simulink model "ModeStatAndRsp_2"  (R2018b)
settings: Solver=FixedStepDiscrete  StartTime=0.0  StopTime=10.0  FixedStep=0.01  RelTol=1e-3
settings Model: Creator=sn2xws  LastModifiedBy=sn2xws
settings ModelReferenceCC: ModelReferenceNumInstancesAllowed=Single

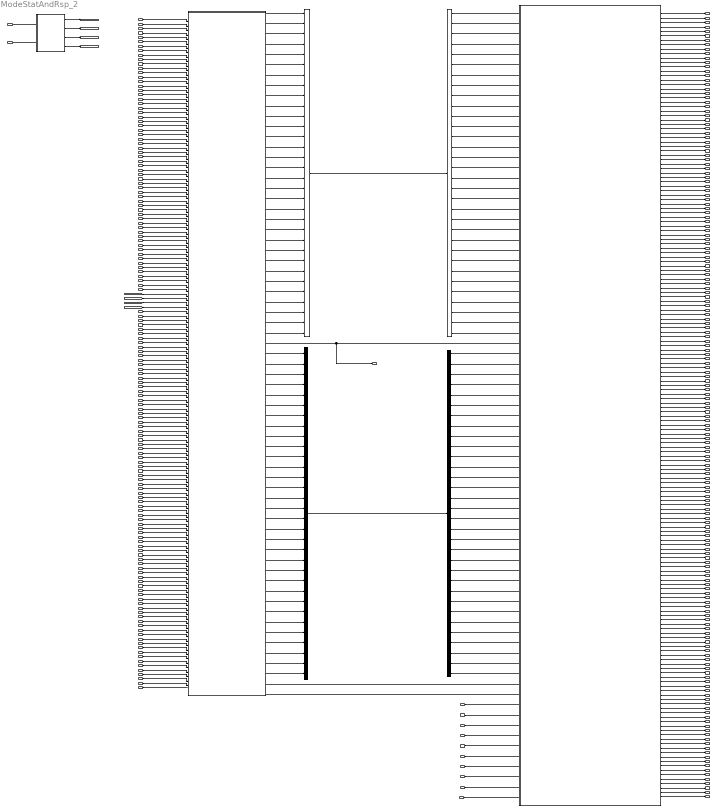
== system ModeStatAndRsp_2 ==
  MdXX_isTrgtPosRunnable : Inport  SampleTime=0.01  OutputFunctionCall=on
  isAcsMdEntryArrivedAtTargetPos_Val : Inport  Port=2  OutDataTypeStr=boolean  PortDimensions=1
  isAcsMdExtArrivedAtTargetPos_Val : Inport  Port=3  OutDataTypeStr=boolean  PortDimensions=1
  isINTMArrivedAtTargetPos_Val : Inport  Port=4  OutDataTypeStr=boolean  PortDimensions=1
  isINTMRArrivedAtTargetPos_Val : Inport  Port=5  OutDataTypeStr=boolean  PortDimensions=1
  isLfFamlyArrivedAtTargetPos_Val : Inport  Port=6  OutDataTypeStr=boolean  PortDimensions=1
  isLfLugArrivedAtTargetPos_Val : Inport  Port=7  OutDataTypeStr=boolean  PortDimensions=1
  isLfLyArrivedAtTargetPos_Val : Inport  Port=8  OutDataTypeStr=boolean  PortDimensions=1
  isLfRecoveryArrivedAtTargetPos_Val : Inport  Port=9  OutDataTypeStr=boolean  PortDimensions=1
  isLfVipArrivedAtTargetPos_Val : Inport  Port=10  OutDataTypeStr=boolean  PortDimensions=1
  isLgrstCloseLArrivedAtTargetPos_Val : Inport  Port=11  OutDataTypeStr=boolean  PortDimensions=1
  isLgrstCloseRArrivedAtTargetPos_Val : Inport  Port=12  OutDataTypeStr=boolean  PortDimensions=1
  isLgrstOpenLArrivedAtTargetPos_Val : Inport  Port=13  OutDataTypeStr=boolean  PortDimensions=1
  isLgrstOpenRArrivedAtTargetPos_Val : Inport  Port=14  OutDataTypeStr=boolean  PortDimensions=1
  isRtFamlyArrivedAtTargetPos_Val : Inport  Port=15  OutDataTypeStr=boolean  PortDimensions=1
  isRtLugArrivedAtTargetPos_Val : Inport  Port=16  OutDataTypeStr=boolean  PortDimensions=1
  isRtLyArrivedAtTargetPos_Val : Inport  Port=17  OutDataTypeStr=boolean  PortDimensions=1
  isRtRecoveryArrivedAtTargetPos_Val : Inport  Port=18  OutDataTypeStr=boolean  PortDimensions=1
  isRtVipArrivedAtTargetPos_Val : Inport  Port=19  OutDataTypeStr=boolean  PortDimensions=1
  MdXX_RspOutCommRunnable : Inport  Port=20  SampleTime=0.01  OutputFunctionCall=on
  MdXX_StatusRunnable : Inport  Port=21  SampleTime=0.01  OutputFunctionCall=on
  StPassCmprtMdHMIDisCmdRunnable : Inport  Port=22  SampleTime=0.01  OutputFunctionCall=on
  PwrMdChked_Val : Inport  Port=23  OutDataTypeStr=Enum: PowerMode1  PortDimensions=1
  CHM2CtrlRunnable : Inport  Port=24  SampleTime=0.01  OutputFunctionCall=on
  IfVeSMSuChmMgrStat_Val : Inport  Port=25  OutDataTypeStr=uint16  PortDimensions=1
  MdXX_StatusToNetWorkRunnable : Inport  Port=26  SampleTime=0.01  OutputFunctionCall=on
  MdXX_RspSelcRunnable : Inport  Port=27  SampleTime=0.01  OutputFunctionCall=on
  SRSModeStateRunnable : Inport  Port=28  SampleTime=0.01  OutputFunctionCall=on
  StNumChkRunnable : Inport  Port=29  SampleTime=0.01  OutputFunctionCall=on
  IfVeSMSeStNumConfig_Val : Inport  Port=30  OutDataTypeStr=Enum: IfVeSMSeStNumConfig  PortDimensions=1
  StateOnOffChkRunnable : Inport  Port=31  SampleTime=0.01  OutputFunctionCall=on
  CommCond_Val : Inport  Port=32  OutDataTypeStr=boolean  PortDimensions=1
  CommExitCond_Val : Inport  Port=33  OutDataTypeStr=boolean  PortDimensions=1
  CommExitCondwithSpeed_Val : Inport  Port=34  OutDataTypeStr=boolean  PortDimensions=1
  isAcsMdEntryDoneFailed_Val : Inport  Port=35  OutDataTypeStr=boolean  PortDimensions=1
  isAcsMdEntryDoneOK_Val : Inport  Port=36  OutDataTypeStr=boolean  PortDimensions=1
  isAcsMdExtDoneFailed_Val : Inport  Port=37  OutDataTypeStr=boolean  PortDimensions=1
  isAcsMdExtDoneOK_Val : Inport  Port=38  OutDataTypeStr=boolean  PortDimensions=1
  isINTMDoneFailed_Val : Inport  Port=39  OutDataTypeStr=boolean  PortDimensions=1
  isINTMDoneOK_Val : Inport  Port=40  OutDataTypeStr=boolean  PortDimensions=1
  isINTMRDoneFailed_Val : Inport  Port=41  OutDataTypeStr=boolean  PortDimensions=1
  isINTMRDoneOK_Val : Inport  Port=42  OutDataTypeStr=boolean  PortDimensions=1
  isLfFamlyDoneFailed_Val : Inport  Port=43  OutDataTypeStr=boolean  PortDimensions=1
  isLfFamlyDoneOK_Val : Inport  Port=44  OutDataTypeStr=boolean  PortDimensions=1
  isLfLugDoneFailed_Val : Inport  Port=45  OutDataTypeStr=boolean  PortDimensions=1
  isLfLugDoneOK_Val : Inport  Port=46  OutDataTypeStr=boolean  PortDimensions=1
  isLfLyDoneFailed_Val : Inport  Port=47  OutDataTypeStr=boolean  PortDimensions=1
  isLfLyDoneOK_Val : Inport  Port=48  OutDataTypeStr=boolean  PortDimensions=1
  isLfRecoveryDoneFailed_Val : Inport  Port=49  OutDataTypeStr=boolean  PortDimensions=1
  isLfRecoveryDoneOK_Val : Inport  Port=50  OutDataTypeStr=boolean  PortDimensions=1
  isLfVipDoneFailed_Val : Inport  Port=51  OutDataTypeStr=boolean  PortDimensions=1
  isLfVipDoneOK_Val : Inport  Port=52  OutDataTypeStr=boolean  PortDimensions=1
  isLgrstCloseLDoneFailed_Val : Inport  Port=53  OutDataTypeStr=boolean  PortDimensions=1
  isLgrstCloseLDoneOK_Val : Inport  Port=54  OutDataTypeStr=boolean  PortDimensions=1
  isLgrstCloseRDoneFailed_Val : Inport  Port=55  OutDataTypeStr=boolean  PortDimensions=1
  isLgrstCloseRDoneOK_Val : Inport  Port=56  OutDataTypeStr=boolean  PortDimensions=1
  isLgrstOpenLDoneFailed_Val : Inport  Port=57  OutDataTypeStr=boolean  PortDimensions=1
  isLgrstOpenLDoneOK_Val : Inport  Port=58  OutDataTypeStr=boolean  PortDimensions=1
  isLgrstOpenRDoneFailed_Val : Inport  Port=59  OutDataTypeStr=boolean  PortDimensions=1
  isLgrstOpenRDoneOK_Val : Inport  Port=60  OutDataTypeStr=boolean  PortDimensions=1
  isRfFamlyDoneFailed_Val : Inport  Port=61  OutDataTypeStr=boolean  PortDimensions=1
  isRfFamlyDoneOK_Val : Inport  Port=62  OutDataTypeStr=boolean  PortDimensions=1
  isRtLugDoneFailed_Val : Inport  Port=63  OutDataTypeStr=boolean  PortDimensions=1
  isRtLugDoneOK_Val : Inport  Port=64  OutDataTypeStr=boolean  PortDimensions=1
  isRtLyDoneFailed_Val : Inport  Port=65  OutDataTypeStr=boolean  PortDimensions=1
  isRtLyDoneOK_Val : Inport  Port=66  OutDataTypeStr=boolean  PortDimensions=1
  isRtRecoveryDoneFailed_Val : Inport  Port=67  OutDataTypeStr=boolean  PortDimensions=1
  isRtRecoveryDoneOK_Val : Inport  Port=68  OutDataTypeStr=boolean  PortDimensions=1
  isRtVipDoneFailed_Val : Inport  Port=69  OutDataTypeStr=boolean  PortDimensions=1
  isRtVipDoneOK_Val : Inport  Port=70  OutDataTypeStr=boolean  PortDimensions=1
  R3LMdSeatOccupied_Val : Inport  Port=71  OutDataTypeStr=boolean  PortDimensions=1
  R3RMdSeatOccupied_Val : Inport  Port=72  OutDataTypeStr=boolean  PortDimensions=1
  SoftIntAcsEnty_Val : Inport  Port=73  OutDataTypeStr=IntEnable  PortDimensions=1
  SoftIntAcsExt_Val : Inport  Port=74  OutDataTypeStr=IntEnable  PortDimensions=1
  SoftIntAllLug_Val : Inport  Port=75  OutDataTypeStr=IntEnable  PortDimensions=1
  SoftIntAllVip_Val : Inport  Port=76  OutDataTypeStr=IntEnable  PortDimensions=1
  SoftIntIntimacyRt_Val : Inport  Port=77  OutDataTypeStr=IntEnable  PortDimensions=1
  SoftIntINTM_Val : Inport  Port=78  OutDataTypeStr=IntEnable  PortDimensions=1
  SoftIntLfFamly_Val : Inport  Port=79  OutDataTypeStr=IntEnable  PortDimensions=1
  SoftIntLfLug_Val : Inport  Port=80  OutDataTypeStr=IntEnable  PortDimensions=1
  SoftIntLfLy_Val : Inport  Port=81  OutDataTypeStr=IntEnable  PortDimensions=1
  SoftIntLfRcvy_Val : Inport  Port=82  OutDataTypeStr=IntEnable  PortDimensions=1
  SoftIntLfVip_Val : Inport  Port=83  OutDataTypeStr=IntEnable  PortDimensions=1
  SoftIntLgrstCloseLt_Val : Inport  Port=84  OutDataTypeStr=IntEnable  PortDimensions=1
  SoftIntLgrstCloseRt_Val : Inport  Port=85  OutDataTypeStr=IntEnable  PortDimensions=1
  SoftIntLgrstOpenLt_Val : Inport  Port=86  OutDataTypeStr=IntEnable  PortDimensions=1
  SoftIntLgrstOpenRt_Val : Inport  Port=87  OutDataTypeStr=IntEnable  PortDimensions=1
  SoftIntRtFamly_Val : Inport  Port=88  OutDataTypeStr=IntEnable  PortDimensions=1
  SoftIntRtLug_Val : Inport  Port=89  OutDataTypeStr=IntEnable  PortDimensions=1
  SoftIntRtLy_Val : Inport  Port=90  OutDataTypeStr=IntEnable  PortDimensions=1
  SoftIntRtRcvy_Val : Inport  Port=91  OutDataTypeStr=IntEnable  PortDimensions=1
  SoftIntRtVip_Val : Inport  Port=92  OutDataTypeStr=IntEnable  PortDimensions=1
  SwIntAcsEnty_Val : Inport  Port=93  OutDataTypeStr=IntEnable  PortDimensions=1
  SwIntAcsExt_Val : Inport  Port=94  OutDataTypeStr=IntEnable  PortDimensions=1
  SwIntAllLug_Val : Inport  Port=95  OutDataTypeStr=IntEnable  PortDimensions=1
  SwIntAllVip_Val : Inport  Port=96  OutDataTypeStr=IntEnable  PortDimensions=1
  SwIntIntimacyRt_Val : Inport  Port=97  OutDataTypeStr=IntEnable  PortDimensions=1
  SwIntINTM_Val : Inport  Port=98  OutDataTypeStr=IntEnable  PortDimensions=1
  SwIntLfFamly_Val : Inport  Port=99  OutDataTypeStr=IntEnable  PortDimensions=1
  SwIntLfLug_Val : Inport  Port=100  OutDataTypeStr=IntEnable  PortDimensions=1
  SwIntLfLy_Val : Inport  Port=101  OutDataTypeStr=IntEnable  PortDimensions=1
  SwIntLfRcvy_Val : Inport  Port=102  OutDataTypeStr=IntEnable  PortDimensions=1
  SwIntLfVip_Val : Inport  Port=103  OutDataTypeStr=IntEnable  PortDimensions=1
  SwIntLgrstCloseLt_Val : Inport  Port=104  OutDataTypeStr=IntEnable  PortDimensions=1
  SwIntLgrstCloseRt_Val : Inport  Port=105  OutDataTypeStr=IntEnable  PortDimensions=1
  SwIntLgrstOpenLt_Val : Inport  Port=106  OutDataTypeStr=IntEnable  PortDimensions=1
  SwIntLgrstOpenRt_Val : Inport  Port=107  OutDataTypeStr=IntEnable  PortDimensions=1
  SwIntRtFamly_Val : Inport  Port=108  OutDataTypeStr=IntEnable  PortDimensions=1
  SwIntRtLug_Val : Inport  Port=109  OutDataTypeStr=IntEnable  PortDimensions=1
  SwIntRtLy_Val : Inport  Port=110  OutDataTypeStr=IntEnable  PortDimensions=1
  SwIntRtRcvy_Val : Inport  Port=111  OutDataTypeStr=IntEnable  PortDimensions=1
  SwIntRtVip_Val : Inport  Port=112  OutDataTypeStr=IntEnable  PortDimensions=1
  MdXX_RspChkRunnable : Inport  Port=113  SampleTime=0.01  OutputFunctionCall=on
  acsEntyMdReq_Val : Inport  Port=114  OutDataTypeStr=boolean  PortDimensions=1
  acsExtMdReq_Val : Inport  Port=115  OutDataTypeStr=boolean  PortDimensions=1
  AllLugMdReq_Val : Inport  Port=116  OutDataTypeStr=boolean  PortDimensions=1
  AllVipMdReq_Val : Inport  Port=117  OutDataTypeStr=boolean  PortDimensions=1
  IntimacyRtMdReq_Val : Inport  Port=118  OutDataTypeStr=boolean  PortDimensions=1
  INTMMdReq_Val : Inport  Port=119  OutDataTypeStr=boolean  PortDimensions=1
  LfFamlyReq_Val : Inport  Port=120  OutDataTypeStr=boolean  PortDimensions=1
  LfLyMdReq_Val : Inport  Port=121  OutDataTypeStr=boolean  PortDimensions=1
  LgrstCloseLtMdReq_Val : Inport  Port=122  OutDataTypeStr=boolean  PortDimensions=1
  LgrstCloseRtMdReq_Val : Inport  Port=123  OutDataTypeStr=boolean  PortDimensions=1
  LgrstOpenLtMdReq_Val : Inport  Port=124  OutDataTypeStr=boolean  PortDimensions=1
  LgrstOpenRtMdReq_Val : Inport  Port=125  OutDataTypeStr=boolean  PortDimensions=1
  LtLugMdReq_Val : Inport  Port=126  OutDataTypeStr=boolean  PortDimensions=1
  LtRcvyMdReq_Val : Inport  Port=127  OutDataTypeStr=boolean  PortDimensions=1
  LtVipMdReq_Val : Inport  Port=128  OutDataTypeStr=boolean  PortDimensions=1
  RtFamlyMdReq_Val : Inport  Port=129  OutDataTypeStr=boolean  PortDimensions=1
  RtLugMdReq_Val : Inport  Port=130  OutDataTypeStr=boolean  PortDimensions=1
  RtLyMdReq_Val : Inport  Port=131  OutDataTypeStr=boolean  PortDimensions=1
  RtRcvyMdReq_Val : Inport  Port=132  OutDataTypeStr=boolean  PortDimensions=1
  RtVipMdReq_Val : Inport  Port=133  OutDataTypeStr=boolean  PortDimensions=1
  LugMdLtAvl_Val : Inport  Port=134  OutDataTypeStr=boolean  PortDimensions=1
  LugMdRtAvl_Val : Inport  Port=135  OutDataTypeStr=boolean  PortDimensions=1
  VipMdLtAvl_Val : Inport  Port=136  OutDataTypeStr=boolean  PortDimensions=1
  VipMdRtAvl_Val : Inport  Port=137  OutDataTypeStr=boolean  PortDimensions=1
  MdEnCtrlAndBsyChkRunnable : Inport  Port=138  SampleTime=0.01  OutputFunctionCall=on
  MdXX_SrcTpRunnable : Inport  Port=139  SampleTime=0.01  OutputFunctionCall=on
  acsEntyMdSrcTp_Val : Inport  Port=140  OutDataTypeStr=Enum: SrcReqTp1  PortDimensions=1
  acsExtMdSrcTp_Val : Inport  Port=141  OutDataTypeStr=Enum: SrcReqTp1  PortDimensions=1
  AllLugSrcReqTp_Val : Inport  Port=142  OutDataTypeStr=Enum: SrcReqTp1  PortDimensions=1
  AllVipSrcReqTp_Val : Inport  Port=143  OutDataTypeStr=Enum: SrcReqTp1  PortDimensions=1
  IntimacyRtMdSrcTp_Val : Inport  Port=144  OutDataTypeStr=Enum: SrcReqTp1  PortDimensions=1
  INTMSrcReqTp_Val : Inport  Port=145  OutDataTypeStr=Enum: SrcReqTp1  PortDimensions=1
  LfFamlySrcReqTp_Val : Inport  Port=146  OutDataTypeStr=Enum: SrcReqTp1  PortDimensions=1
  LfLySrcReqTp_Val : Inport  Port=147  OutDataTypeStr=Enum: SrcReqTp1  PortDimensions=1
  LgrstCloseLtSrcReqTp_Val : Inport  Port=148  OutDataTypeStr=Enum: SrcReqTp1  PortDimensions=1
  LgrstCloseRtSrcReqTp_Val : Inport  Port=149  OutDataTypeStr=Enum: SrcReqTp1  PortDimensions=1
  LgrstOpenLtSrcReqTp_Val : Inport  Port=150  OutDataTypeStr=Enum: SrcReqTp1  PortDimensions=1
  LgrstOpenRtSrcReqTp_Val : Inport  Port=151  OutDataTypeStr=Enum: SrcReqTp1  PortDimensions=1
  LtLugSrcReqTp_Val : Inport  Port=152  OutDataTypeStr=Enum: SrcReqTp1  PortDimensions=1
  LtRcvySrcReqTp_Val : Inport  Port=153  OutDataTypeStr=Enum: SrcReqTp1  PortDimensions=1
  LtVipSrcReqTp_Val : Inport  Port=154  OutDataTypeStr=Enum: SrcReqTp1  PortDimensions=1
  RtFamlySrcReqTp_Val : Inport  Port=155  OutDataTypeStr=Enum: SrcReqTp1  PortDimensions=1
  RtLugSrcReqTp_Val : Inport  Port=156  OutDataTypeStr=Enum: SrcReqTp1  PortDimensions=1
  RtLySrcReqTp_Val : Inport  Port=157  OutDataTypeStr=Enum: SrcReqTp1  PortDimensions=1
  RtRcvySrcReqTp_Val : Inport  Port=158  OutDataTypeStr=Enum: SrcReqTp1  PortDimensions=1
  RtVipSrcReqTp_Val : Inport  Port=159  OutDataTypeStr=Enum: SrcReqTp1  PortDimensions=1
  PosArray_Val : Inport  Port=160  OutDataTypeStr=uint8  PortDimensions=11
  Demux : Demux  Outputs=32
  Demux1 : Demux  Outputs=32
  Model : ModelReference  ModelNameDialog=StNumChk.slx  SimulationMode=Normal  ModelReferenceVersion=V2.0.0
  Model1 : ModelReference  ModelNameDialog=ModeStatCtrl.slx  SimulationMode=Normal  ModelReferenceVersion=1.27
  Model3 : ModelReference  ModelNameDialog=ModeRsp.slx  SimulationMode=Normal  ModelReferenceVersion=1.35
  Mux : Mux  Inputs=32
  Mux1 : Mux  Inputs=32
  IfVeSMSuStPassCmprtMdHMIDisCmd_Val : Outport  OutDataTypeStr=uint8  PortDimensions=1
  IfVeSMSeStPassCmprtMdNoti2ChmEvntStat_Val : Outport  Port=2  OutDataTypeStr=Enum: EventSts1  PortDimensions=1
  IfVeSMSeStPassCmprtMdCrtMdStat_Val : Outport  Port=3  OutDataTypeStr=uint8  PortDimensions=1
  IfVeSMSuStPassCmprtMd_Md1_CrtStat_Val : Outport  Port=4  OutDataTypeStr=uint8  PortDimensions=1
  IfVeSMSuStPassCmprtMd_Md10_CrtStat_Val : Outport  Port=5  OutDataTypeStr=uint8  PortDimensions=1
  IfVeSMSuStPassCmprtMd_Md11_CrtStat_Val : Outport  Port=6  OutDataTypeStr=uint8  PortDimensions=1
  IfVeSMSuStPassCmprtMd_Md12_CrtStat_Val : Outport  Port=7  OutDataTypeStr=uint8  PortDimensions=1
  IfVeSMSuStPassCmprtMd_Md13_CrtStat_Val : Outport  Port=8  OutDataTypeStr=uint8  PortDimensions=1
  IfVeSMSuStPassCmprtMd_Md14_CrtStat_Val : Outport  Port=9  OutDataTypeStr=uint8  PortDimensions=1
  IfVeSMSuStPassCmprtMd_Md15_CrtStat_Val : Outport  Port=10  OutDataTypeStr=uint8  PortDimensions=1
  IfVeSMSuStPassCmprtMd_Md16_CrtStat_Val : Outport  Port=11  OutDataTypeStr=uint8  PortDimensions=1
  IfVeSMSuStPassCmprtMd_Md17_CrtStat_Val : Outport  Port=12  OutDataTypeStr=uint8  PortDimensions=1
  IfVeSMSuStPassCmprtMd_Md18_CrtStat_Val : Outport  Port=13  OutDataTypeStr=uint8  PortDimensions=1
  IfVeSMSuStPassCmprtMd_Md19_CrtStat_Val : Outport  Port=14  OutDataTypeStr=uint8  PortDimensions=1
  IfVeSMSuStPassCmprtMd_Md2_CrtStat_Val : Outport  Port=15  OutDataTypeStr=uint8  PortDimensions=1
  IfVeSMSuStPassCmprtMd_Md20_CrtStat_Val : Outport  Port=16  OutDataTypeStr=uint8  PortDimensions=1
  IfVeSMSuStPassCmprtMd_Md21_CrtStat_Val : Outport  Port=17  OutDataTypeStr=uint8  PortDimensions=1
  IfVeSMSuStPassCmprtMd_Md22_CrtStat_Val : Outport  Port=18  OutDataTypeStr=uint8  PortDimensions=1
  IfVeSMSuStPassCmprtMd_Md23_CrtStat_Val : Outport  Port=19  OutDataTypeStr=uint8  PortDimensions=1
  IfVeSMSuStPassCmprtMd_Md24_CrtStat_Val : Outport  Port=20  OutDataTypeStr=uint8  PortDimensions=1
  IfVeSMSuStPassCmprtMd_Md25_CrtStat_Val : Outport  Port=21  OutDataTypeStr=uint8  PortDimensions=1
  IfVeSMSuStPassCmprtMd_Md26_CrtStat_Val : Outport  Port=22  OutDataTypeStr=uint8  PortDimensions=1
  IfVeSMSuStPassCmprtMd_Md27_CrtStat_Val : Outport  Port=23  OutDataTypeStr=uint8  PortDimensions=1
  IfVeSMSuStPassCmprtMd_Md28_CrtStat_Val : Outport  Port=24  OutDataTypeStr=uint8  PortDimensions=1
  IfVeSMSuStPassCmprtMd_Md29_CrtStat_Val : Outport  Port=25  OutDataTypeStr=uint8  PortDimensions=1
  IfVeSMSuStPassCmprtMd_Md3_CrtStat_Val : Outport  Port=26  OutDataTypeStr=uint8  PortDimensions=1
  IfVeSMSuStPassCmprtMd_Md30_CrtStat_Val : Outport  Port=27  OutDataTypeStr=uint8  PortDimensions=1
  IfVeSMSuStPassCmprtMd_Md31_CrtStat_Val : Outport  Port=28  OutDataTypeStr=uint8  PortDimensions=1
  IfVeSMSuStPassCmprtMd_Md32_CrtStat_Val : Outport  Port=29  OutDataTypeStr=uint8  PortDimensions=1
  IfVeSMSuStPassCmprtMd_Md4_CrtStat_Val : Outport  Port=30  OutDataTypeStr=uint8  PortDimensions=1
  IfVeSMSuStPassCmprtMd_Md5_CrtStat_Val : Outport  Port=31  OutDataTypeStr=uint8  PortDimensions=1
  IfVeSMSuStPassCmprtMd_Md6_CrtStat_Val : Outport  Port=32  OutDataTypeStr=uint8  PortDimensions=1
  IfVeSMSuStPassCmprtMd_Md7_CrtStat_Val : Outport  Port=33  OutDataTypeStr=uint8  PortDimensions=1
  IfVeSMSuStPassCmprtMd_Md8_CrtStat_Val : Outport  Port=34  OutDataTypeStr=uint8  PortDimensions=1
  IfVeSMSuStPassCmprtMd_Md9_CrtStat_Val : Outport  Port=35  OutDataTypeStr=uint8  PortDimensions=1
  IfVeSMSuSRSCrt_MdSw1_Stat_Val : Outport  Port=36  OutDataTypeStr=uint8  PortDimensions=1
  IfVeSMSuSRSCrt_MdSw10_Stat_Val : Outport  Port=37  OutDataTypeStr=uint8  PortDimensions=1
  IfVeSMSuSRSCrt_MdSw2_Stat_Val : Outport  Port=38  OutDataTypeStr=uint8  PortDimensions=1
  IfVeSMSuSRSCrt_MdSw3_Stat_Val : Outport  Port=39  OutDataTypeStr=uint8  PortDimensions=1
  IfVeSMSuSRSCrt_MdSw4_Stat_Val : Outport  Port=40  OutDataTypeStr=uint8  PortDimensions=1
  IfVeSMSuSRSCrt_MdSw5_Stat_Val : Outport  Port=41  OutDataTypeStr=uint8  PortDimensions=1
  IfVeSMSuSRSCrt_MdSw6_Stat_Val : Outport  Port=42  OutDataTypeStr=uint8  PortDimensions=1
  IfVeSMSuSRSCrt_MdSw7_Stat_Val : Outport  Port=43  OutDataTypeStr=uint8  PortDimensions=1
  IfVeSMSuSRSCrt_MdSw8_Stat_Val : Outport  Port=44  OutDataTypeStr=uint8  PortDimensions=1
  IfVeSMSuSRSCrt_MdSw9_Stat_Val : Outport  Port=45  OutDataTypeStr=uint8  PortDimensions=1
  IfVeSMSuSRSCrtMdIndTyp_67_2_Val : Outport  Port=46  OutDataTypeStr=uint8  PortDimensions=1
  IfVeSMStPassCmprtMd_RfCtrl_Sw_RclRspStat_Val : Outport  Port=47  OutDataTypeStr=uint8  PortDimensions=1
  IfVeSMSuHMI2L_StMd1_Rsp_Val : Outport  Port=48  OutDataTypeStr=uint8  PortDimensions=1
  IfVeSMSuHMI2L_StMd10_Rsp_Val : Outport  Port=49  OutDataTypeStr=uint8  PortDimensions=1
  IfVeSMSuHMI2L_StMd11_Rsp_Val : Outport  Port=50  OutDataTypeStr=uint8  PortDimensions=1
  IfVeSMSuHMI2L_StMd12_Rsp_Val : Outport  Port=51  OutDataTypeStr=uint8  PortDimensions=1
  IfVeSMSuHMI2L_StMd13_Rsp_Val : Outport  Port=52  OutDataTypeStr=uint8  PortDimensions=1
  IfVeSMSuHMI2L_StMd14_Rsp_Val : Outport  Port=53  OutDataTypeStr=uint8  PortDimensions=1
  IfVeSMSuHMI2L_StMd15_Rsp_Val : Outport  Port=54  OutDataTypeStr=uint8  PortDimensions=1
  IfVeSMSuHMI2L_StMd16_Rsp_Val : Outport  Port=55  OutDataTypeStr=uint8  PortDimensions=1
  IfVeSMSuHMI2L_StMd17_Rsp_Val : Outport  Port=56  OutDataTypeStr=uint8  PortDimensions=1
  IfVeSMSuHMI2L_StMd18_Rsp_Val : Outport  Port=57  OutDataTypeStr=uint8  PortDimensions=1
  IfVeSMSuHMI2L_StMd19_Rsp_Val : Outport  Port=58  OutDataTypeStr=uint8  PortDimensions=1
  IfVeSMSuHMI2L_StMd2_Rsp_Val : Outport  Port=59  OutDataTypeStr=uint8  PortDimensions=1
  IfVeSMSuHMI2L_StMd20_Rsp_Val : Outport  Port=60  OutDataTypeStr=uint8  PortDimensions=1
  IfVeSMSuHMI2L_StMd21_Rsp_Val : Outport  Port=61  OutDataTypeStr=uint8  PortDimensions=1
  IfVeSMSuHMI2L_StMd22_Rsp_Val : Outport  Port=62  OutDataTypeStr=uint8  PortDimensions=1
  IfVeSMSuHMI2L_StMd23_Rsp_Val : Outport  Port=63  OutDataTypeStr=uint8  PortDimensions=1
  IfVeSMSuHMI2L_StMd24_Rsp_Val : Outport  Port=64  OutDataTypeStr=uint8  PortDimensions=1
  IfVeSMSuHMI2L_StMd25_Rsp_Val : Outport  Port=65  OutDataTypeStr=uint8  PortDimensions=1
  IfVeSMSuHMI2L_StMd26_Rsp_Val : Outport  Port=66  OutDataTypeStr=uint8  PortDimensions=1
  IfVeSMSuHMI2L_StMd27_Rsp_Val : Outport  Port=67  OutDataTypeStr=uint8  PortDimensions=1
  IfVeSMSuHMI2L_StMd28_Rsp_Val : Outport  Port=68  OutDataTypeStr=uint8  PortDimensions=1
  IfVeSMSuHMI2L_StMd29_Rsp_Val : Outport  Port=69  OutDataTypeStr=uint8  PortDimensions=1
  IfVeSMSuHMI2L_StMd3_Rsp_Val : Outport  Port=70  OutDataTypeStr=uint8  PortDimensions=1
  IfVeSMSuHMI2L_StMd30_Rsp_Val : Outport  Port=71  OutDataTypeStr=uint8  PortDimensions=1
  IfVeSMSuHMI2L_StMd31_Rsp_Val : Outport  Port=72  OutDataTypeStr=uint8  PortDimensions=1
  IfVeSMSuHMI2L_StMd32_Rsp_Val : Outport  Port=73  OutDataTypeStr=uint8  PortDimensions=1
  IfVeSMSuHMI2L_StMd4_Rsp_Val : Outport  Port=74  OutDataTypeStr=uint8  PortDimensions=1
  IfVeSMSuHMI2L_StMd5_Rsp_Val : Outport  Port=75  OutDataTypeStr=uint8  PortDimensions=1
  IfVeSMSuHMI2L_StMd6_Rsp_Val : Outport  Port=76  OutDataTypeStr=uint8  PortDimensions=1
  IfVeSMSuHMI2L_StMd7_Rsp_Val : Outport  Port=77  OutDataTypeStr=uint8  PortDimensions=1
  IfVeSMSuHMI2L_StMd8_Rsp_Val : Outport  Port=78  OutDataTypeStr=uint8  PortDimensions=1
  IfVeSMSuHMI2L_StMd9_Rsp_Val : Outport  Port=79  OutDataTypeStr=uint8  PortDimensions=1
  IfVeSMSuHMI2R_StMd1_Rsp_Val : Outport  Port=80  OutDataTypeStr=uint8  PortDimensions=1
  IfVeSMSuHMI2R_StMd10_Rsp_Val : Outport  Port=81  OutDataTypeStr=uint8  PortDimensions=1
  IfVeSMSuHMI2R_StMd11_Rsp_Val : Outport  Port=82  OutDataTypeStr=uint8  PortDimensions=1
  IfVeSMSuHMI2R_StMd12_Rsp_Val : Outport  Port=83  OutDataTypeStr=uint8  PortDimensions=1
  IfVeSMSuHMI2R_StMd13_Rsp_Val : Outport  Port=84  OutDataTypeStr=uint8  PortDimensions=1
  IfVeSMSuHMI2R_StMd14_Rsp_Val : Outport  Port=85  OutDataTypeStr=uint8  PortDimensions=1
  IfVeSMSuHMI2R_StMd15_Rsp_Val : Outport  Port=86  OutDataTypeStr=uint8  PortDimensions=1
  IfVeSMSuHMI2R_StMd16_Rsp_Val : Outport  Port=87  OutDataTypeStr=uint8  PortDimensions=1
  IfVeSMSuHMI2R_StMd17_Rsp_Val : Outport  Port=88  OutDataTypeStr=uint8  PortDimensions=1
  IfVeSMSuHMI2R_StMd18_Rsp_Val : Outport  Port=89  OutDataTypeStr=uint8  PortDimensions=1
  IfVeSMSuHMI2R_StMd19_Rsp_Val : Outport  Port=90  OutDataTypeStr=uint8  PortDimensions=1
  IfVeSMSuHMI2R_StMd2_Rsp_Val : Outport  Port=91  OutDataTypeStr=uint8  PortDimensions=1
  IfVeSMSuHMI2R_StMd20_Rsp_Val : Outport  Port=92  OutDataTypeStr=uint8  PortDimensions=1
  IfVeSMSuHMI2R_StMd21_Rsp_Val : Outport  Port=93  OutDataTypeStr=uint8  PortDimensions=1
  IfVeSMSuHMI2R_StMd22_Rsp_Val : Outport  Port=94  OutDataTypeStr=uint8  PortDimensions=1
  IfVeSMSuHMI2R_StMd23_Rsp_Val : Outport  Port=95  OutDataTypeStr=uint8  PortDimensions=1
  IfVeSMSuHMI2R_StMd24_Rsp_Val : Outport  Port=96  OutDataTypeStr=uint8  PortDimensions=1
  IfVeSMSuHMI2R_StMd25_Rsp_Val : Outport  Port=97  OutDataTypeStr=uint8  PortDimensions=1
  IfVeSMSuHMI2R_StMd26_Rsp_Val : Outport  Port=98  OutDataTypeStr=uint8  PortDimensions=1
  IfVeSMSuHMI2R_StMd27_Rsp_Val : Outport  Port=99  OutDataTypeStr=uint8  PortDimensions=1
  IfVeSMSuHMI2R_StMd28_Rsp_Val : Outport  Port=100  OutDataTypeStr=uint8  PortDimensions=1
  IfVeSMSuHMI2R_StMd29_Rsp_Val : Outport  Port=101  OutDataTypeStr=uint8  PortDimensions=1
  IfVeSMSuHMI2R_StMd3_Rsp_Val : Outport  Port=102  OutDataTypeStr=uint8  PortDimensions=1
  IfVeSMSuHMI2R_StMd30_Rsp_Val : Outport  Port=103  OutDataTypeStr=uint8  PortDimensions=1
  IfVeSMSuHMI2R_StMd31_Rsp_Val : Outport  Port=104  OutDataTypeStr=uint8  PortDimensions=1
  IfVeSMSuHMI2R_StMd32_Rsp_Val : Outport  Port=105  OutDataTypeStr=uint8  PortDimensions=1
  IfVeSMSuHMI2R_StMd4_Rsp_Val : Outport  Port=106  OutDataTypeStr=uint8  PortDimensions=1
  IfVeSMSuHMI2R_StMd5_Rsp_Val : Outport  Port=107  OutDataTypeStr=uint8  PortDimensions=1
  IfVeSMSuHMI2R_StMd6_Rsp_Val : Outport  Port=108  OutDataTypeStr=uint8  PortDimensions=1
  IfVeSMSuHMI2R_StMd7_Rsp_Val : Outport  Port=109  OutDataTypeStr=uint8  PortDimensions=1
  IfVeSMSuHMI2R_StMd8_Rsp_Val : Outport  Port=110  OutDataTypeStr=uint8  PortDimensions=1
  IfVeSMSuHMI2R_StMd9_Rsp_Val : Outport  Port=111  OutDataTypeStr=uint8  PortDimensions=1
  IfVeSMSuStPassCmprtMd10RclRspStat_Val : Outport  Port=112  OutDataTypeStr=uint8  PortDimensions=1
  IfVeSMSuStPassCmprtMd11RclRspStat_Val : Outport  Port=113  OutDataTypeStr=uint8  PortDimensions=1
  IfVeSMSuStPassCmprtMd12RclRspStat_Val : Outport  Port=114  OutDataTypeStr=uint8  PortDimensions=1
  IfVeSMSuStPassCmprtMd13RclRspStat_Val : Outport  Port=115  OutDataTypeStr=uint8  PortDimensions=1
  IfVeSMSuStPassCmprtMd14RclRspStat_Val : Outport  Port=116  OutDataTypeStr=uint8  PortDimensions=1
  IfVeSMSuStPassCmprtMd15RclRspStat_Val : Outport  Port=117  OutDataTypeStr=uint8  PortDimensions=1
  IfVeSMSuStPassCmprtMd16RclRspStat_Val : Outport  Port=118  OutDataTypeStr=uint8  PortDimensions=1
  IfVeSMSuStPassCmprtMd17RclRspStat_Val : Outport  Port=119  OutDataTypeStr=uint8  PortDimensions=1
  IfVeSMSuStPassCmprtMd18RclRspStat_Val : Outport  Port=120  OutDataTypeStr=uint8  PortDimensions=1
  IfVeSMSuStPassCmprtMd19RclRspStat_Val : Outport  Port=121  OutDataTypeStr=uint8  PortDimensions=1
  IfVeSMSuStPassCmprtMd1RclRspStat_Val : Outport  Port=122  OutDataTypeStr=uint8  PortDimensions=1
  IfVeSMSuStPassCmprtMd20RclRspStat_Val : Outport  Port=123  OutDataTypeStr=uint8  PortDimensions=1
  IfVeSMSuStPassCmprtMd21RclRspStat_Val : Outport  Port=124  OutDataTypeStr=uint8  PortDimensions=1
  IfVeSMSuStPassCmprtMd22RclRspStat_Val : Outport  Port=125  OutDataTypeStr=uint8  PortDimensions=1
  IfVeSMSuStPassCmprtMd23RclRspStat_Val : Outport  Port=126  OutDataTypeStr=uint8  PortDimensions=1
  IfVeSMSuStPassCmprtMd24RclRspStat_Val : Outport  Port=127  OutDataTypeStr=uint8  PortDimensions=1
  IfVeSMSuStPassCmprtMd25RclRspStat_Val : Outport  Port=128  OutDataTypeStr=uint8  PortDimensions=1
  IfVeSMSuStPassCmprtMd26RclRspStat_Val : Outport  Port=129  OutDataTypeStr=uint8  PortDimensions=1
  IfVeSMSuStPassCmprtMd27RclRspStat_Val : Outport  Port=130  OutDataTypeStr=uint8  PortDimensions=1
  IfVeSMSuStPassCmprtMd28RclRspStat_Val : Outport  Port=131  OutDataTypeStr=uint8  PortDimensions=1
  IfVeSMSuStPassCmprtMd29RclRspStat_Val : Outport  Port=132  OutDataTypeStr=uint8  PortDimensions=1
  IfVeSMSuStPassCmprtMd2RclRspStat_Val : Outport  Port=133  OutDataTypeStr=uint8  PortDimensions=1
  IfVeSMSuStPassCmprtMd30RclRspStat_Val : Outport  Port=134  OutDataTypeStr=uint8  PortDimensions=1
  IfVeSMSuStPassCmprtMd31RclRspStat_Val : Outport  Port=135  OutDataTypeStr=uint8  PortDimensions=1
  IfVeSMSuStPassCmprtMd32RclRspStat_Val : Outport  Port=136  OutDataTypeStr=uint8  PortDimensions=1
  IfVeSMSuStPassCmprtMd3RclRspStat_Val : Outport  Port=137  OutDataTypeStr=uint8  PortDimensions=1
  IfVeSMSuStPassCmprtMd4RclRspStat_Val : Outport  Port=138  OutDataTypeStr=uint8  PortDimensions=1
  IfVeSMSuStPassCmprtMd5RclRspStat_Val : Outport  Port=139  OutDataTypeStr=uint8  PortDimensions=1
  IfVeSMSuStPassCmprtMd6RclRspStat_Val : Outport  Port=140  OutDataTypeStr=uint8  PortDimensions=1
  IfVeSMSuStPassCmprtMd7RclRspStat_Val : Outport  Port=141  OutDataTypeStr=uint8  PortDimensions=1
  IfVeSMSuStPassCmprtMd8RclRspStat_Val : Outport  Port=142  OutDataTypeStr=uint8  PortDimensions=1
  IfVeSMSuStPassCmprtMd9RclRspStat_Val : Outport  Port=143  OutDataTypeStr=uint8  PortDimensions=1
  IfVeSMSuStSrv_StMd1_Rsp_Val : Outport  Port=144  OutDataTypeStr=uint8  PortDimensions=1
  IfVeSMSuStSrv_StMd10_Rsp_Val : Outport  Port=145  OutDataTypeStr=uint8  PortDimensions=1
  IfVeSMSuStSrv_StMd11_Rsp_Val : Outport  Port=146  OutDataTypeStr=uint8  PortDimensions=1
  IfVeSMSuStSrv_StMd12_Rsp_Val : Outport  Port=147  OutDataTypeStr=uint8  PortDimensions=1
  IfVeSMSuStSrv_StMd13_Rsp_Val : Outport  Port=148  OutDataTypeStr=uint8  PortDimensions=1
  IfVeSMSuStSrv_StMd14_Rsp_Val : Outport  Port=149  OutDataTypeStr=uint8  PortDimensions=1
  IfVeSMSuStSrv_StMd15_Rsp_Val : Outport  Port=150  OutDataTypeStr=uint8  PortDimensions=1
  IfVeSMSuStSrv_StMd16_Rsp_Val : Outport  Port=151  OutDataTypeStr=uint8  PortDimensions=1
  IfVeSMSuStSrv_StMd17_Rsp_Val : Outport  Port=152  OutDataTypeStr=uint8  PortDimensions=1
  IfVeSMSuStSrv_StMd18_Rsp_Val : Outport  Port=153  OutDataTypeStr=uint8  PortDimensions=1
  IfVeSMSuStSrv_StMd19_Rsp_Val : Outport  Port=154  OutDataTypeStr=uint8  PortDimensions=1
  IfVeSMSuStSrv_StMd2_Rsp_Val : Outport  Port=155  OutDataTypeStr=uint8  PortDimensions=1
  IfVeSMSuStSrv_StMd20_Rsp_Val : Outport  Port=156  OutDataTypeStr=uint8  PortDimensions=1
  IfVeSMSuStSrv_StMd21_Rsp_Val : Outport  Port=157  OutDataTypeStr=uint8  PortDimensions=1
  IfVeSMSuStSrv_StMd22_Rsp_Val : Outport  Port=158  OutDataTypeStr=uint8  PortDimensions=1
  IfVeSMSuStSrv_StMd23_Rsp_Val : Outport  Port=159  OutDataTypeStr=uint8  PortDimensions=1
  IfVeSMSuStSrv_StMd24_Rsp_Val : Outport  Port=160  OutDataTypeStr=uint8  PortDimensions=1
  IfVeSMSuStSrv_StMd25_Rsp_Val : Outport  Port=161  OutDataTypeStr=uint8  PortDimensions=1
  IfVeSMSuStSrv_StMd26_Rsp_Val : Outport  Port=162  OutDataTypeStr=uint8  PortDimensions=1
  IfVeSMSuStSrv_StMd27_Rsp_Val : Outport  Port=163  OutDataTypeStr=uint8  PortDimensions=1
  IfVeSMSuStSrv_StMd28_Rsp_Val : Outport  Port=164  OutDataTypeStr=uint8  PortDimensions=1
  IfVeSMSuStSrv_StMd29_Rsp_Val : Outport  Port=165  OutDataTypeStr=uint8  PortDimensions=1
  IfVeSMSuStSrv_StMd3_Rsp_Val : Outport  Port=166  OutDataTypeStr=uint8  PortDimensions=1
  IfVeSMSuStSrv_StMd30_Rsp_Val : Outport  Port=167  OutDataTypeStr=uint8  PortDimensions=1
  IfVeSMSuStSrv_StMd31_Rsp_Val : Outport  Port=168  OutDataTypeStr=uint8  PortDimensions=1
  IfVeSMSuStSrv_StMd32_Rsp_Val : Outport  Port=169  OutDataTypeStr=uint8  PortDimensions=1
  IfVeSMSuStSrv_StMd4_Rsp_Val : Outport  Port=170  OutDataTypeStr=uint8  PortDimensions=1
  IfVeSMSuStSrv_StMd5_Rsp_Val : Outport  Port=171  OutDataTypeStr=uint8  PortDimensions=1
  IfVeSMSuStSrv_StMd6_Rsp_Val : Outport  Port=172  OutDataTypeStr=uint8  PortDimensions=1
  IfVeSMSuStSrv_StMd7_Rsp_Val : Outport  Port=173  OutDataTypeStr=uint8  PortDimensions=1
  IfVeSMSuStSrv_StMd8_Rsp_Val : Outport  Port=174  OutDataTypeStr=uint8  PortDimensions=1
  IfVeSMSuStSrv_StMd9_Rsp_Val : Outport  Port=175  OutDataTypeStr=uint8  PortDimensions=1
  oModeState_Val : Outport  Port=176  OutDataTypeStr=Enum: MdTp1  PortDimensions=1
  SRSMode_Val : Outport  Port=177  OutDataTypeStr=Enum: SRSCurMode1  PortDimensions=1
  ModeSrcTpLt_Val : Outport  Port=178  OutDataTypeStr=Enum: SrcReqTp1  PortDimensions=1
  modestate32_Val : Outport  Port=179  OutDataTypeStr=uint32  PortDimensions=1
  wires:
  MdXX_isTrgtPosRunnable/1 -> Model1/134
  isAcsMdEntryArrivedAtTargetPos_Val/1 -> Model1/135
  isAcsMdExtArrivedAtTargetPos_Val/1 -> Model1/136
  isINTMArrivedAtTargetPos_Val/1 -> Model1/137
  isINTMRArrivedAtTargetPos_Val/1 -> Model1/138
  isLfFamlyArrivedAtTargetPos_Val/1 -> Model1/139
  isLfLugArrivedAtTargetPos_Val/1 -> Model1/140
  isLfLyArrivedAtTargetPos_Val/1 -> Model1/141
  isLfRecoveryArrivedAtTargetPos_Val/1 -> Model1/142
  isLfVipArrivedAtTargetPos_Val/1 -> Model1/143
  isLgrstCloseLArrivedAtTargetPos_Val/1 -> Model1/144
  isLgrstCloseRArrivedAtTargetPos_Val/1 -> Model1/145
  isLgrstOpenLArrivedAtTargetPos_Val/1 -> Model1/146
  isLgrstOpenRArrivedAtTargetPos_Val/1 -> Model1/147
  isRtFamlyArrivedAtTargetPos_Val/1 -> Model1/148
  isRtLugArrivedAtTargetPos_Val/1 -> Model1/149
  isRtLyArrivedAtTargetPos_Val/1 -> Model1/150
  isRtRecoveryArrivedAtTargetPos_Val/1 -> Model1/151
  isRtVipArrivedAtTargetPos_Val/1 -> ?
  Model1/7 -> Mux/7
  Model1/6 -> Mux/6
  Model1/8 -> Mux/8
  Model1/5 -> Mux/5
  Model1/9 -> Mux/9
  Model1/4 -> Mux/4
  Model1/10 -> Mux/10
  Model1/3 -> Mux/3
  Model1/11 -> Mux/11
  Model1/2 -> Mux/2
  Model1/12 -> Mux/12
  Model1/1 -> Mux/1
  Model1/13 -> Mux/13
  Model1/14 -> Mux/14
  Model1/15 -> Mux/15
  Model1/16 -> Mux/16
  Model1/17 -> Mux/17
  Model1/18 -> Mux/18
  Model1/19 -> Mux/19
  Model1/20 -> Mux/20
  Model1/21 -> Mux/21
  Model1/22 -> Mux/22
  Model1/23 -> Mux/23
  Model1/24 -> Mux/24
  Model1/25 -> Mux/25
  Model1/26 -> Mux/26
  Model1/27 -> Mux/27
  Model1/28 -> Mux/28
  Model1/29 -> Mux/29
  Model1/30 -> Mux/30
  Model1/31 -> Mux/31
  Model1/32 -> Mux/32
  Model1/33 -> modestate32_Val/1, Model3/33
  Mux/1 -> Demux/1
  Mux1/1 -> Demux1/1
  StNumChkRunnable/1 -> Model/1
  IfVeSMSeStNumConfig_Val/1 -> Model/2
  Model/1 -> [StNumFlg_Is4s]
  Model/4 -> [StNumFlg_Is7s]
  Model/3 -> [StNumFlg_Is6s7s]
  Model/2 -> [StNumFlg_Is6s]
  StateOnOffChkRunnable/1 -> Model1/1
  CommCond_Val/1 -> Model1/2
  CommExitCond_Val/1 -> Model1/3
  CommExitCondwithSpeed_Val/1 -> Model1/4
  isAcsMdEntryDoneFailed_Val/1 -> Model1/5
  isAcsMdEntryDoneOK_Val/1 -> Model1/6
  isAcsMdExtDoneFailed_Val/1 -> Model1/7
  isAcsMdExtDoneOK_Val/1 -> Model1/8
  isINTMDoneFailed_Val/1 -> Model1/9
  isINTMDoneOK_Val/1 -> Model1/10
  isINTMRDoneFailed_Val/1 -> Model1/11
  isINTMRDoneOK_Val/1 -> Model1/12
  isLfFamlyDoneFailed_Val/1 -> Model1/13
  isLfFamlyDoneOK_Val/1 -> Model1/14
  isLfLugDoneFailed_Val/1 -> Model1/15
  isLfLugDoneOK_Val/1 -> Model1/16
  isLfLyDoneFailed_Val/1 -> Model1/17
  isLfLyDoneOK_Val/1 -> Model1/18
  isLfRecoveryDoneFailed_Val/1 -> Model1/19
  isLfRecoveryDoneOK_Val/1 -> Model1/20
  isLfVipDoneFailed_Val/1 -> Model1/21
  isLfVipDoneOK_Val/1 -> Model1/22
  isLgrstCloseLDoneFailed_Val/1 -> Model1/23
  isLgrstCloseLDoneOK_Val/1 -> Model1/24
  isLgrstCloseRDoneFailed_Val/1 -> Model1/25
  isLgrstCloseRDoneOK_Val/1 -> Model1/26
  isLgrstOpenLDoneFailed_Val/1 -> Model1/27
  isLgrstOpenLDoneOK_Val/1 -> Model1/28
  isLgrstOpenRDoneFailed_Val/1 -> Model1/29
  isLgrstOpenRDoneOK_Val/1 -> Model1/30
  isRfFamlyDoneFailed_Val/1 -> Model1/31
  isRfFamlyDoneOK_Val/1 -> Model1/32
  isRtLugDoneFailed_Val/1 -> Model1/33
  isRtLugDoneOK_Val/1 -> Model1/34
  isRtLyDoneFailed_Val/1 -> Model1/35
  isRtLyDoneOK_Val/1 -> Model1/36
  isRtRecoveryDoneFailed_Val/1 -> Model1/37
  isRtRecoveryDoneOK_Val/1 -> Model1/38
  isRtVipDoneFailed_Val/1 -> Model1/39
  isRtVipDoneOK_Val/1 -> Model1/40
  R3LMdSeatOccupied_Val/1 -> Model1/41
  R3RMdSeatOccupied_Val/1 -> Model1/42
  SoftIntAcsEnty_Val/1 -> Model1/43
  SoftIntAcsExt_Val/1 -> Model1/44
  SoftIntAllLug_Val/1 -> Model1/45
  SoftIntAllVip_Val/1 -> Model1/46
  SoftIntIntimacyRt_Val/1 -> Model1/47
  SoftIntINTM_Val/1 -> Model1/48
  SoftIntLfFamly_Val/1 -> Model1/49
  SoftIntLfLug_Val/1 -> Model1/50
  SoftIntLfLy_Val/1 -> Model1/51
  SoftIntLfRcvy_Val/1 -> Model1/52
  SoftIntLfVip_Val/1 -> Model1/53
  SoftIntLgrstCloseLt_Val/1 -> Model1/54
  SoftIntLgrstCloseRt_Val/1 -> Model1/55
  SoftIntLgrstOpenLt_Val/1 -> Model1/56
  SoftIntLgrstOpenRt_Val/1 -> Model1/57
  SoftIntRtFamly_Val/1 -> Model1/58
  SoftIntRtLug_Val/1 -> Model1/59
  SoftIntRtLy_Val/1 -> Model1/60
  SoftIntRtRcvy_Val/1 -> Model1/61
  SoftIntRtVip_Val/1 -> Model1/62
  [StNumFlg_Is4s] -> Model1/63
  [StNumFlg_Is6s] -> Model1/64
  [StNumFlg_Is6s7s] -> Model1/65
  [StNumFlg_Is7s] -> Model1/66
  SwIntAcsEnty_Val/1 -> Model1/67
  SwIntAcsExt_Val/1 -> Model1/68
  SwIntAllLug_Val/1 -> Model1/69
  SwIntAllVip_Val/1 -> Model1/70
  SwIntIntimacyRt_Val/1 -> Model1/71
  SwIntINTM_Val/1 -> Model1/72
  SwIntLfFamly_Val/1 -> Model1/73
  SwIntLfLug_Val/1 -> Model1/74
  SwIntLfLy_Val/1 -> Model1/75
  SwIntLfRcvy_Val/1 -> Model1/76
  SwIntLfVip_Val/1 -> Model1/77
  SwIntLgrstCloseLt_Val/1 -> Model1/78
  SwIntLgrstCloseRt_Val/1 -> Model1/79
  SwIntLgrstOpenLt_Val/1 -> Model1/80
  SwIntLgrstOpenRt_Val/1 -> Model1/81
  SwIntRtFamly_Val/1 -> Model1/82
  SwIntRtLug_Val/1 -> Model1/83
  SwIntRtLy_Val/1 -> Model1/84
  SwIntRtRcvy_Val/1 -> Model1/85
  SwIntRtVip_Val/1 -> Model1/86
  MdXX_RspChkRunnable/1 -> Model1/87
  acsEntyMdReq_Val/1 -> Model1/88
  acsExtMdReq_Val/1 -> Model1/89
  AllLugMdReq_Val/1 -> Model1/90
  AllVipMdReq_Val/1 -> Model1/91
  IntimacyRtMdReq_Val/1 -> Model1/92
  INTMMdReq_Val/1 -> Model1/93
  LfFamlyReq_Val/1 -> Model1/94
  LfLyMdReq_Val/1 -> Model1/95
  LgrstCloseLtMdReq_Val/1 -> Model1/96
  LgrstCloseRtMdReq_Val/1 -> Model1/97
  LgrstOpenLtMdReq_Val/1 -> Model1/98
  LgrstOpenRtMdReq_Val/1 -> Model1/99
  LtLugMdReq_Val/1 -> Model1/100
  LtRcvyMdReq_Val/1 -> Model1/101
  LtVipMdReq_Val/1 -> Model1/102
  RtFamlyMdReq_Val/1 -> Model1/103
  RtLugMdReq_Val/1 -> Model1/104
  RtLyMdReq_Val/1 -> Model1/105
  RtRcvyMdReq_Val/1 -> Model1/106
  RtVipMdReq_Val/1 -> Model1/107
  LugMdLtAvl_Val/1 -> Model1/108
  LugMdRtAvl_Val/1 -> Model1/109
  VipMdLtAvl_Val/1 -> Model1/110
  VipMdRtAvl_Val/1 -> Model1/111
  MdEnCtrlAndBsyChkRunnable/1 -> Model1/112
  MdXX_SrcTpRunnable/1 -> Model1/113
  acsEntyMdSrcTp_Val/1 -> Model1/114
  acsExtMdSrcTp_Val/1 -> Model1/115
  AllLugSrcReqTp_Val/1 -> Model1/116
  AllVipSrcReqTp_Val/1 -> Model1/117
  IntimacyRtMdSrcTp_Val/1 -> Model1/118
  INTMSrcReqTp_Val/1 -> Model1/119
  LfFamlySrcReqTp_Val/1 -> Model1/120
  LfLySrcReqTp_Val/1 -> Model1/121
  LgrstCloseLtSrcReqTp_Val/1 -> Model1/122
  LgrstCloseRtSrcReqTp_Val/1 -> Model1/123
  LgrstOpenLtSrcReqTp_Val/1 -> Model1/124
  LgrstOpenRtSrcReqTp_Val/1 -> Model1/125
  LtLugSrcReqTp_Val/1 -> Model1/126
  LtRcvySrcReqTp_Val/1 -> Model1/127
  LtVipSrcReqTp_Val/1 -> Model1/128
  RtFamlySrcReqTp_Val/1 -> Model1/129
  RtLugSrcReqTp_Val/1 -> Model1/130
  RtLySrcReqTp_Val/1 -> Model1/131
  RtRcvySrcReqTp_Val/1 -> Model1/132
  RtVipSrcReqTp_Val/1 -> Model1/133
  Model3/1 -> IfVeSMSuStPassCmprtMdHMIDisCmd_Val/1
  Model3/2 -> IfVeSMSeStPassCmprtMdNoti2ChmEvntStat_Val/1
  Model3/3 -> IfVeSMSeStPassCmprtMdCrtMdStat_Val/1
  Model3/4 -> IfVeSMSuStPassCmprtMd_Md1_CrtStat_Val/1
  Model3/5 -> IfVeSMSuStPassCmprtMd_Md10_CrtStat_Val/1
  Model3/6 -> IfVeSMSuStPassCmprtMd_Md11_CrtStat_Val/1
  Model3/7 -> IfVeSMSuStPassCmprtMd_Md12_CrtStat_Val/1
  Model3/8 -> IfVeSMSuStPassCmprtMd_Md13_CrtStat_Val/1
  Model3/9 -> IfVeSMSuStPassCmprtMd_Md14_CrtStat_Val/1
  Model3/10 -> IfVeSMSuStPassCmprtMd_Md15_CrtStat_Val/1
  Model3/11 -> IfVeSMSuStPassCmprtMd_Md16_CrtStat_Val/1
  Model3/12 -> IfVeSMSuStPassCmprtMd_Md17_CrtStat_Val/1
  Model3/13 -> IfVeSMSuStPassCmprtMd_Md18_CrtStat_Val/1
  Model3/14 -> IfVeSMSuStPassCmprtMd_Md19_CrtStat_Val/1
  Model3/15 -> IfVeSMSuStPassCmprtMd_Md2_CrtStat_Val/1
  Model3/16 -> IfVeSMSuStPassCmprtMd_Md20_CrtStat_Val/1
  Model3/17 -> IfVeSMSuStPassCmprtMd_Md21_CrtStat_Val/1
  Model3/18 -> IfVeSMSuStPassCmprtMd_Md22_CrtStat_Val/1
  Model3/19 -> IfVeSMSuStPassCmprtMd_Md23_CrtStat_Val/1
  Model3/20 -> IfVeSMSuStPassCmprtMd_Md24_CrtStat_Val/1
  Model3/21 -> IfVeSMSuStPassCmprtMd_Md25_CrtStat_Val/1
  Model3/22 -> IfVeSMSuStPassCmprtMd_Md26_CrtStat_Val/1
  Model3/23 -> IfVeSMSuStPassCmprtMd_Md27_CrtStat_Val/1
  Model3/24 -> IfVeSMSuStPassCmprtMd_Md28_CrtStat_Val/1
  Model3/25 -> IfVeSMSuStPassCmprtMd_Md29_CrtStat_Val/1
  Model3/26 -> IfVeSMSuStPassCmprtMd_Md3_CrtStat_Val/1
  Model3/27 -> IfVeSMSuStPassCmprtMd_Md30_CrtStat_Val/1
  Model3/28 -> IfVeSMSuStPassCmprtMd_Md31_CrtStat_Val/1
  Model3/29 -> IfVeSMSuStPassCmprtMd_Md32_CrtStat_Val/1
  Model3/30 -> IfVeSMSuStPassCmprtMd_Md4_CrtStat_Val/1
  Model3/31 -> IfVeSMSuStPassCmprtMd_Md5_CrtStat_Val/1
  Model3/32 -> IfVeSMSuStPassCmprtMd_Md6_CrtStat_Val/1
  Model3/33 -> IfVeSMSuStPassCmprtMd_Md7_CrtStat_Val/1
  Model3/34 -> IfVeSMSuStPassCmprtMd_Md8_CrtStat_Val/1
  Model3/35 -> IfVeSMSuStPassCmprtMd_Md9_CrtStat_Val/1
  Model3/36 -> IfVeSMSuSRSCrt_MdSw1_Stat_Val/1
  Model3/37 -> IfVeSMSuSRSCrt_MdSw10_Stat_Val/1
  Model3/38 -> IfVeSMSuSRSCrt_MdSw2_Stat_Val/1
  Model3/39 -> IfVeSMSuSRSCrt_MdSw3_Stat_Val/1
  Model3/40 -> IfVeSMSuSRSCrt_MdSw4_Stat_Val/1
  Model3/41 -> IfVeSMSuSRSCrt_MdSw5_Stat_Val/1
  Model3/42 -> IfVeSMSuSRSCrt_MdSw6_Stat_Val/1
  Model3/43 -> IfVeSMSuSRSCrt_MdSw7_Stat_Val/1
  Model3/44 -> IfVeSMSuSRSCrt_MdSw8_Stat_Val/1
  Model3/45 -> IfVeSMSuSRSCrt_MdSw9_Stat_Val/1
  Model3/46 -> IfVeSMSuSRSCrtMdIndTyp_67_2_Val/1
  Model3/47 -> IfVeSMStPassCmprtMd_RfCtrl_Sw_RclRspStat_Val/1
  Model3/48 -> IfVeSMSuHMI2L_StMd1_Rsp_Val/1
  Model3/49 -> IfVeSMSuHMI2L_StMd10_Rsp_Val/1
  Model3/50 -> IfVeSMSuHMI2L_StMd11_Rsp_Val/1
  Model3/51 -> IfVeSMSuHMI2L_StMd12_Rsp_Val/1
  Model3/52 -> IfVeSMSuHMI2L_StMd13_Rsp_Val/1
  Model3/53 -> IfVeSMSuHMI2L_StMd14_Rsp_Val/1
  Model3/54 -> IfVeSMSuHMI2L_StMd15_Rsp_Val/1
  Model3/55 -> IfVeSMSuHMI2L_StMd16_Rsp_Val/1
  Model3/56 -> IfVeSMSuHMI2L_StMd17_Rsp_Val/1
  Model3/57 -> IfVeSMSuHMI2L_StMd18_Rsp_Val/1
  Model3/58 -> IfVeSMSuHMI2L_StMd19_Rsp_Val/1
  Model3/59 -> IfVeSMSuHMI2L_StMd2_Rsp_Val/1
  Model3/60 -> IfVeSMSuHMI2L_StMd20_Rsp_Val/1
  Model3/61 -> IfVeSMSuHMI2L_StMd21_Rsp_Val/1
  Model3/62 -> IfVeSMSuHMI2L_StMd22_Rsp_Val/1
  Model3/63 -> IfVeSMSuHMI2L_StMd23_Rsp_Val/1
  Model3/64 -> IfVeSMSuHMI2L_StMd24_Rsp_Val/1
  Model3/65 -> IfVeSMSuHMI2L_StMd25_Rsp_Val/1
  Model3/66 -> IfVeSMSuHMI2L_StMd26_Rsp_Val/1
  Model3/67 -> IfVeSMSuHMI2L_StMd27_Rsp_Val/1
  Model3/68 -> IfVeSMSuHMI2L_StMd28_Rsp_Val/1
  Model3/69 -> IfVeSMSuHMI2L_StMd29_Rsp_Val/1
  Model3/70 -> IfVeSMSuHMI2L_StMd3_Rsp_Val/1
  Model3/71 -> IfVeSMSuHMI2L_StMd30_Rsp_Val/1
  Model3/72 -> IfVeSMSuHMI2L_StMd31_Rsp_Val/1
  Model3/73 -> IfVeSMSuHMI2L_StMd32_Rsp_Val/1
  Model3/74 -> IfVeSMSuHMI2L_StMd4_Rsp_Val/1
  Model3/75 -> IfVeSMSuHMI2L_StMd5_Rsp_Val/1
  Model3/76 -> IfVeSMSuHMI2L_StMd6_Rsp_Val/1
  Model3/77 -> IfVeSMSuHMI2L_StMd7_Rsp_Val/1
  Model3/78 -> IfVeSMSuHMI2L_StMd8_Rsp_Val/1
  Model3/79 -> IfVeSMSuHMI2L_StMd9_Rsp_Val/1
  Model3/80 -> IfVeSMSuHMI2R_StMd1_Rsp_Val/1
  Model3/81 -> IfVeSMSuHMI2R_StMd10_Rsp_Val/1
  Model3/82 -> IfVeSMSuHMI2R_StMd11_Rsp_Val/1
  Model3/83 -> IfVeSMSuHMI2R_StMd12_Rsp_Val/1
  Model3/84 -> IfVeSMSuHMI2R_StMd13_Rsp_Val/1
  Model3/85 -> IfVeSMSuHMI2R_StMd14_Rsp_Val/1
  Model3/86 -> IfVeSMSuHMI2R_StMd15_Rsp_Val/1
  Model3/87 -> IfVeSMSuHMI2R_StMd16_Rsp_Val/1
  Model3/88 -> IfVeSMSuHMI2R_StMd17_Rsp_Val/1
  Model3/89 -> IfVeSMSuHMI2R_StMd18_Rsp_Val/1
  Model3/90 -> IfVeSMSuHMI2R_StMd19_Rsp_Val/1
  Model3/91 -> IfVeSMSuHMI2R_StMd2_Rsp_Val/1
  Model3/92 -> IfVeSMSuHMI2R_StMd20_Rsp_Val/1
  Model3/93 -> IfVeSMSuHMI2R_StMd21_Rsp_Val/1
  Model3/94 -> IfVeSMSuHMI2R_StMd22_Rsp_Val/1
  Model3/95 -> IfVeSMSuHMI2R_StMd23_Rsp_Val/1
  Model3/96 -> IfVeSMSuHMI2R_StMd24_Rsp_Val/1
  Model3/97 -> IfVeSMSuHMI2R_StMd25_Rsp_Val/1
  Model3/98 -> IfVeSMSuHMI2R_StMd26_Rsp_Val/1
  Model3/99 -> IfVeSMSuHMI2R_StMd27_Rsp_Val/1
  Model3/100 -> IfVeSMSuHMI2R_StMd28_Rsp_Val/1
  Model3/101 -> IfVeSMSuHMI2R_StMd29_Rsp_Val/1
  Model3/102 -> IfVeSMSuHMI2R_StMd3_Rsp_Val/1
  Model3/103 -> IfVeSMSuHMI2R_StMd30_Rsp_Val/1
  Model3/104 -> IfVeSMSuHMI2R_StMd31_Rsp_Val/1
  Model3/105 -> IfVeSMSuHMI2R_StMd32_Rsp_Val/1
  Model3/106 -> IfVeSMSuHMI2R_StMd4_Rsp_Val/1
  Model3/107 -> IfVeSMSuHMI2R_StMd5_Rsp_Val/1
  Model3/108 -> IfVeSMSuHMI2R_StMd6_Rsp_Val/1
  Model3/109 -> IfVeSMSuHMI2R_StMd7_Rsp_Val/1
  Model3/110 -> IfVeSMSuHMI2R_StMd8_Rsp_Val/1
  Model3/111 -> IfVeSMSuHMI2R_StMd9_Rsp_Val/1
  Model3/112 -> IfVeSMSuStPassCmprtMd10RclRspStat_Val/1
  Model3/113 -> IfVeSMSuStPassCmprtMd11RclRspStat_Val/1
  Model3/114 -> IfVeSMSuStPassCmprtMd12RclRspStat_Val/1
  Model3/115 -> IfVeSMSuStPassCmprtMd13RclRspStat_Val/1
  Model3/116 -> IfVeSMSuStPassCmprtMd14RclRspStat_Val/1
  Model3/117 -> IfVeSMSuStPassCmprtMd15RclRspStat_Val/1
  Model3/118 -> IfVeSMSuStPassCmprtMd16RclRspStat_Val/1
  Model3/119 -> IfVeSMSuStPassCmprtMd17RclRspStat_Val/1
  Model3/120 -> IfVeSMSuStPassCmprtMd18RclRspStat_Val/1
  Model3/121 -> IfVeSMSuStPassCmprtMd19RclRspStat_Val/1
  Model3/122 -> IfVeSMSuStPassCmprtMd1RclRspStat_Val/1
  Model3/123 -> IfVeSMSuStPassCmprtMd20RclRspStat_Val/1
  Model3/124 -> IfVeSMSuStPassCmprtMd21RclRspStat_Val/1
  Model3/125 -> IfVeSMSuStPassCmprtMd22RclRspStat_Val/1
  Model3/126 -> IfVeSMSuStPassCmprtMd23RclRspStat_Val/1
  Model3/127 -> IfVeSMSuStPassCmprtMd24RclRspStat_Val/1
  Model3/128 -> IfVeSMSuStPassCmprtMd25RclRspStat_Val/1
  Model3/129 -> IfVeSMSuStPassCmprtMd26RclRspStat_Val/1
  Model3/130 -> IfVeSMSuStPassCmprtMd27RclRspStat_Val/1
  Model3/131 -> IfVeSMSuStPassCmprtMd28RclRspStat_Val/1
  Model3/132 -> IfVeSMSuStPassCmprtMd29RclRspStat_Val/1
  Model3/133 -> IfVeSMSuStPassCmprtMd2RclRspStat_Val/1
  Model3/134 -> IfVeSMSuStPassCmprtMd30RclRspStat_Val/1
  Model3/135 -> IfVeSMSuStPassCmprtMd31RclRspStat_Val/1
  Model3/136 -> IfVeSMSuStPassCmprtMd32RclRspStat_Val/1
  Model3/137 -> IfVeSMSuStPassCmprtMd3RclRspStat_Val/1
  Model3/138 -> IfVeSMSuStPassCmprtMd4RclRspStat_Val/1
  Model3/139 -> IfVeSMSuStPassCmprtMd5RclRspStat_Val/1
  Model3/140 -> IfVeSMSuStPassCmprtMd6RclRspStat_Val/1
  Model3/141 -> IfVeSMSuStPassCmprtMd7RclRspStat_Val/1
  Model3/142 -> IfVeSMSuStPassCmprtMd8RclRspStat_Val/1
  Model3/143 -> IfVeSMSuStPassCmprtMd9RclRspStat_Val/1
  Model3/144 -> IfVeSMSuStSrv_StMd1_Rsp_Val/1
  Model3/145 -> IfVeSMSuStSrv_StMd10_Rsp_Val/1
  Model3/146 -> IfVeSMSuStSrv_StMd11_Rsp_Val/1
  Model3/147 -> IfVeSMSuStSrv_StMd12_Rsp_Val/1
  Model3/148 -> IfVeSMSuStSrv_StMd13_Rsp_Val/1
  Model3/149 -> IfVeSMSuStSrv_StMd14_Rsp_Val/1
  Model3/150 -> IfVeSMSuStSrv_StMd15_Rsp_Val/1
  Model3/151 -> IfVeSMSuStSrv_StMd16_Rsp_Val/1
  Model3/152 -> IfVeSMSuStSrv_StMd17_Rsp_Val/1
  Model3/153 -> IfVeSMSuStSrv_StMd18_Rsp_Val/1
  Model3/154 -> IfVeSMSuStSrv_StMd19_Rsp_Val/1
  Model3/155 -> IfVeSMSuStSrv_StMd2_Rsp_Val/1
  Model3/156 -> IfVeSMSuStSrv_StMd20_Rsp_Val/1
  Model3/157 -> IfVeSMSuStSrv_StMd21_Rsp_Val/1
  Model3/158 -> IfVeSMSuStSrv_StMd22_Rsp_Val/1
  Model3/159 -> IfVeSMSuStSrv_StMd23_Rsp_Val/1
  Model3/160 -> IfVeSMSuStSrv_StMd24_Rsp_Val/1
  Model3/161 -> IfVeSMSuStSrv_StMd25_Rsp_Val/1
  Model3/162 -> IfVeSMSuStSrv_StMd26_Rsp_Val/1
  Model3/163 -> IfVeSMSuStSrv_StMd27_Rsp_Val/1
  Model3/164 -> IfVeSMSuStSrv_StMd28_Rsp_Val/1
  Model3/165 -> IfVeSMSuStSrv_StMd29_Rsp_Val/1
  Model3/166 -> IfVeSMSuStSrv_StMd3_Rsp_Val/1
  Model3/167 -> IfVeSMSuStSrv_StMd30_Rsp_Val/1
  Model3/168 -> IfVeSMSuStSrv_StMd31_Rsp_Val/1
  Model3/169 -> IfVeSMSuStSrv_StMd32_Rsp_Val/1
  Model3/170 -> IfVeSMSuStSrv_StMd4_Rsp_Val/1
  Model3/171 -> IfVeSMSuStSrv_StMd5_Rsp_Val/1
  Model3/172 -> IfVeSMSuStSrv_StMd6_Rsp_Val/1
  Model3/173 -> IfVeSMSuStSrv_StMd7_Rsp_Val/1
  Model3/174 -> IfVeSMSuStSrv_StMd8_Rsp_Val/1
  Model3/175 -> IfVeSMSuStSrv_StMd9_Rsp_Val/1
  Model3/176 -> oModeState_Val/1
  Model3/177 -> SRSMode_Val/1
  Model3/178 -> ModeSrcTpLt_Val/1
  MdXX_StatusToNetWorkRunnable/1 -> Model3/77
  Model1/67 -> Model3/67
  Model1/34 -> Mux1/1
  Model1/35 -> Mux1/2
  Model1/36 -> Mux1/3
  Model1/37 -> Mux1/4
  Model1/38 -> Mux1/5
  Model1/39 -> Mux1/6
  Model1/40 -> Mux1/7
  Model1/41 -> Mux1/8
  Model1/42 -> Mux1/9
  Model1/43 -> Mux1/10
  Model1/44 -> Mux1/11
  Model1/45 -> Mux1/12
  Model1/46 -> Mux1/13
  Model1/47 -> Mux1/14
  Model1/48 -> Mux1/15
  Model1/49 -> Mux1/16
  Model1/50 -> Mux1/17
  Model1/51 -> Mux1/18
  Model1/52 -> Mux1/19
  Model1/53 -> Mux1/20
  Model1/54 -> Mux1/21
  Model1/55 -> Mux1/22
  Model1/56 -> Mux1/23
  Model1/57 -> Mux1/24
  Model1/58 -> Mux1/25
  Model1/59 -> Mux1/26
  Model1/60 -> Mux1/27
  Model1/61 -> Mux1/28
  Model1/62 -> Mux1/29
  Model1/63 -> Mux1/30
  Model1/64 -> Mux1/31
  Model1/65 -> Mux1/32
  Model1/66 -> Model3/66
  Demux/1 -> Model3/1
  Demux/2 -> Model3/2
  Demux/3 -> Model3/3
  Demux/4 -> Model3/4
  Demux/5 -> Model3/5
  Demux/6 -> Model3/6
  Demux/7 -> Model3/7
  Demux/8 -> Model3/8
  Demux/9 -> Model3/9
  Demux/10 -> Model3/10
  Demux/11 -> Model3/11
  Demux/12 -> Model3/12
  Demux/13 -> Model3/13
  Demux/14 -> Model3/14
  Demux/15 -> Model3/15
  Demux/16 -> Model3/16
  Demux/17 -> Model3/17
  Demux/18 -> Model3/18
  Demux/19 -> Model3/19
  Demux/20 -> Model3/20
  Demux/21 -> Model3/21
  Demux/22 -> Model3/22
  Demux/23 -> Model3/23
  Demux/24 -> Model3/24
  Demux/25 -> Model3/25
  Demux/26 -> Model3/26
  Demux/27 -> Model3/27
  Demux/28 -> Model3/28
  Demux/29 -> Model3/29
  Demux/30 -> Model3/30
  Demux/31 -> Model3/31
  Demux/32 -> Model3/32
  Demux1/6 -> Model3/39
  Demux1/5 -> Model3/38
  Demux1/7 -> Model3/40
  Demux1/4 -> Model3/37
  Demux1/8 -> Model3/41
  Demux1/3 -> Model3/36
  Demux1/9 -> Model3/42
  Demux1/2 -> Model3/35
  Demux1/10 -> Model3/43
  Demux1/1 -> Model3/34
  Demux1/11 -> Model3/44
  Demux1/12 -> Model3/45
  Demux1/13 -> Model3/46
  Demux1/14 -> Model3/47
  Demux1/15 -> Model3/48
  Demux1/16 -> Model3/49
  Demux1/17 -> Model3/50
  Demux1/18 -> Model3/51
  Demux1/19 -> Model3/52
  Demux1/20 -> Model3/53
  Demux1/21 -> Model3/54
  Demux1/22 -> Model3/55
  Demux1/23 -> Model3/56
  Demux1/24 -> Model3/57
  Demux1/25 -> Model3/58
  Demux1/26 -> Model3/59
  Demux1/27 -> Model3/60
  Demux1/28 -> Model3/61
  Demux1/29 -> Model3/62
  Demux1/30 -> Model3/63
  Demux1/31 -> Model3/64
  Demux1/32 -> Model3/65
  MdXX_RspOutCommRunnable/1 -> Model3/68
  MdXX_StatusRunnable/1 -> Model3/69
  StPassCmprtMdHMIDisCmdRunnable/1 -> Model3/70
  PwrMdChked_Val/1 -> Model3/71
  CHM2CtrlRunnable/1 -> Model3/72
  IfVeSMSuChmMgrStat_Val/1 -> Model3/73
  MdXX_RspSelcRunnable/1 -> Model3/74
  PosArray_Val/1 -> Model3/75
  SRSModeStateRunnable/1 -> Model3/76
